simulink model "mech_body_driver"  (Simulink 6.0)
settings: Solver=ode45  StartTime=0.0  StopTime=inf  RelTol=1e-3
libraries: mblibv1 x12
settings Model: Creator=dkennedy  LastModifiedBy=batserve  ExtModeAutoUpdateStatusClock=off
settings DataIOCC: SignalLoggingName=sigsOut
settings OptimizationCC: BooleanDataType=off
settings DebuggingCC: CheckExecutionContextPreStartOutputMsg=on  CheckExecutionContextRuntimeOutputMsg=on  SolverPrmCheckMsg=none
settings HardwareCC: TargetUnknown=on
settings SimMechanicsCC: VisOnUpdateDiagram=on  VisDuringSimulation=on

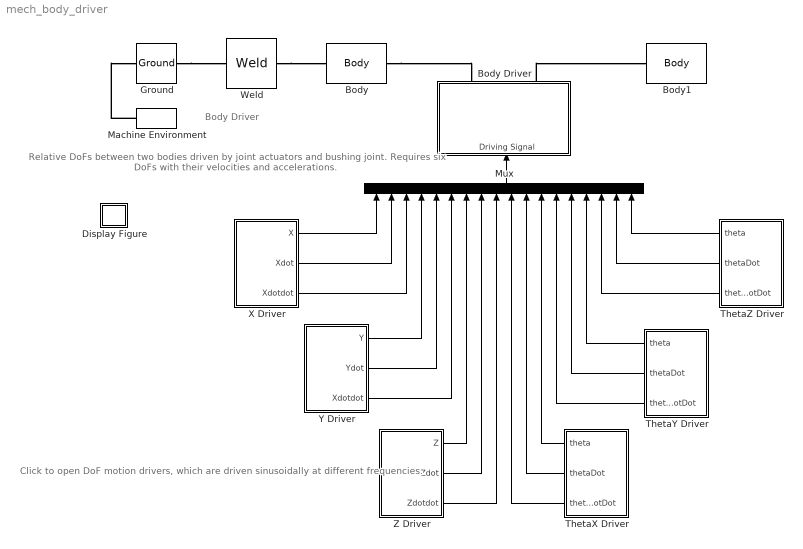
== system mech_body_driver ==
  note: Body Driver
  note: Relative DoFs between two bodies driven by
      | joint actuators and bushing joint. Requires six DoFs with
      | their velocities and accelerations.
  note: Click to open DoF motion drivers,
      | which are driven sinusoidally at
      | different frequencies.
  Body : mblibv1/Bodies/Body  PhysicalDomain=mechanical  SubClassName=Unknown  LeftPortType=workingframe  RightPortType=workingframe  LConnTagsString=CS1  RConnTagsString=CS2  DialogClass=MechanicalBodyBlock  Mass=1  MassUnits=kg  InertiaUnits=kg*m^2  Inertia=0.25*eye(3)  Shape=Cylinder  ShapeDims=[1 1]  ShapeUnits=m  ShapeUse=false  Density=1  DensityUnits=kg/m^3  DensityUse=false  CG=Left$CG$[0 0 0]$WORLD$WORLD$m$[0 0 0]$Euler X-Y-Z$deg$WORLD$false  WorkingFrames=Left$CS1$[0 0 0]$CG$CG$m$[0 0 0]$Euler X-Y-Z$deg$WORLD$true#Right$CS2$[0 0 0]$CG$CG$m$[0 0 0]$Euler X-Y-Z$deg$WORLD$true
  Body Driver : Subsystem  Orientation=up
  Body1 : mblibv1/Bodies/Body  PhysicalDomain=mechanical  SubClassName=Unknown  LeftPortType=workingframe  RightPortType=workingframe  LConnTagsString=CS1  DialogClass=MechanicalBodyBlock  Mass=1  MassUnits=kg  InertiaUnits=kg*m^2  Inertia=[1.5 0 0; 0 1.0 0; 0 0 2.0]  Shape=Cylinder  ShapeDims=[1 1]  ShapeUnits=m  ShapeUse=false  Density=1  DensityUnits=kg/m^3  DensityUse=false  CG=Left$CG$[1 1 1]$WORLD$WORLD$m$[0 0 0]$Euler X-Y-Z$deg$WORLD$false  WorkingFrames=Left$CS1$[0 0 0]$CG$CG$m$[0 0 0]$Euler X-Y-Z$deg$WORLD$true
  Display Figure : Subsystem  Tag=Help  Description="Help callback for body driver model: mech_body_driver.  Opens Help browser to Type 19 marker at documentation for this tutorial model."
      settings: OpenFcn=pmhelpview([docroot '/toolbox/physmod/mech/mech.map'], 'mech_body_driver_help');
      mask Type: Help callback
      mask Display: image(imread('info.bmp'))
  Ground : mblibv1/Bodies/Ground  Opaque=on  LeftPortType=env  RightPortType=workingframe  PhysicalDomain=Mechanical  DialogClass=GroundBlock  CoordPosition=[0 0 0]  CoordPositionUnits=m  StateVectorMgrId=-1  MachineId=[0 0]  ShowEnvPort=on
  Machine Environment : mblibv1/Bodies/Machine Environment  Tag=Factory ground  Orientation=left  DialogController=MECH.DialogSource  Opaque=on  PortType=env  PhysicalDomain=Mechanical  DialogTemplateClass=MECH.MachineEnvironment  SyncWhenCopied=off  Gravity=[0 0 0]  GravityUnits=m/s^2  GravityAsSignal=off  Dimensionality=3D Only  AnalysisType=Forward dynamics  LinearAssemblyTolerance=1e-3  LinearAssemblyToleranceUnits=m  AngularAssemblyTolerance=1e-3  AngularAssemblyToleranceUnits=rad  ConstraintSolverType=Stabilizing  ConstraintRelTolerance=1e-4  ConstraintAbsTolerance=1e-4  UseRobustSingularityHandling=off  StatePerturbationType=Fixed  PerturbationSize=1e-5  VisualizeMachine=on
  Mux : Mux  Orientation=up  Inputs=18
  ThetaX Driver : Subsystem  Orientation=left
  ThetaY Driver : Subsystem  Orientation=left
  ThetaZ Driver : Subsystem  Orientation=left
  Weld : mblibv1/Joints/Weld  PhysicalDomain=mechanical  SubClassName=Unknown  LeftPortType=blob  RightPortType=blob  LConnTagsString=__newl0  RConnTagsString=__newr0  NumSAPorts=0  CutJoint=off  MarkAsCut=off  Primitives=weld  PrimitiveProps=W$INERTIAL$[0 0 0]$weld  DialogClass=JointBlock
  X Driver : Subsystem
  Y Driver : Subsystem
  Z Driver : Subsystem
  wires:
  Mux/1 -> Body Driver/1(Driving Signal)
  X Driver/1(X) -> Mux/1
  X Driver/2(Xdot) -> Mux/2
  X Driver/3(Xdotdot) -> Mux/3
  Y Driver/1(Y) -> Mux/4
  Y Driver/2(Ydot) -> Mux/5
  Y Driver/3(Xdotdot) -> Mux/6
  Z Driver/1(Z) -> Mux/7
  Z Driver/2(Zdot) -> Mux/8
  Z Driver/3(Zdotdot) -> Mux/9
  ThetaX Driver/3(thetaDotDot) -> Mux/10
  ThetaX Driver/2(thetaDot) -> Mux/11
  ThetaX Driver/1(theta) -> Mux/12
  ThetaY Driver/3(thetaDotDot) -> Mux/13
  ThetaY Driver/2(thetaDot) -> Mux/14
  ThetaY Driver/1(theta) -> Mux/15
  ThetaZ Driver/3(thetaDotDot) -> Mux/16
  ThetaZ Driver/2(thetaDot) -> Mux/17
  ThetaZ Driver/1(theta) -> Mux/18
  connections:
  Ground/RConn1 -- Weld/LConn1
  Weld/RConn1 -- Body/LConn1
  Body/RConn1 -- Body Driver/RConn1
  Body Driver/RConn2 -- Body1/LConn1
  Machine Environment/RConn1 -- Ground/LConn1

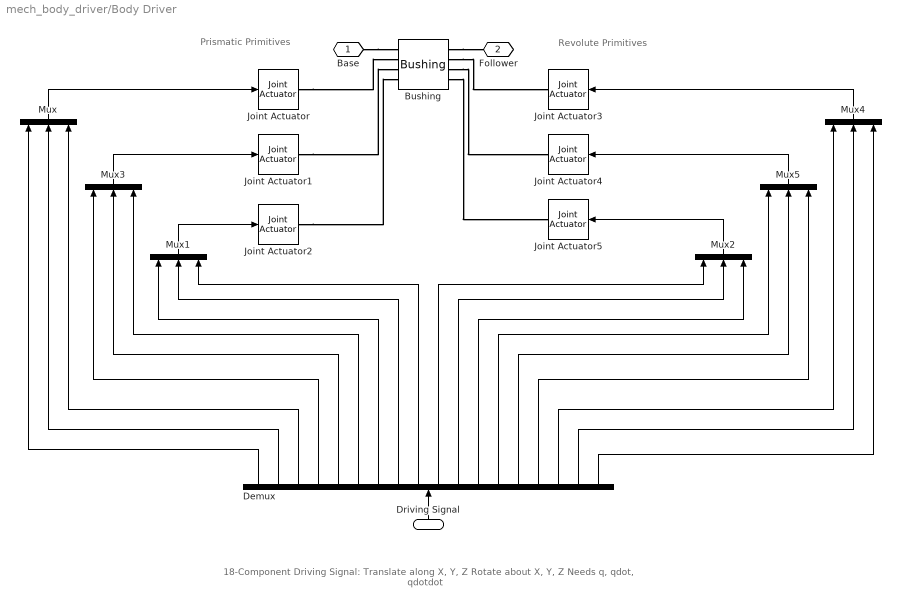
== system mech_body_driver/Body Driver ==
  note: Prismatic Primitives
  note: Revolute Primitives
  note: 18-Component Driving Signal:
      | Translate along X, Y, Z
      | Rotate about X, Y, Z
      | Needs q, qdot, qdotdot
  Driving Signal : Inport  Orientation=up  Port=1  LatchInput=off
  Bushing : mblibv1/Joints/Bushing  PhysicalDomain=mechanical  SubClassName=Unknown  LeftPortType=blob  RightPortType=blob  LConnTagsString=__newl0|SA1|SA2|SA3  RConnTagsString=__newr0|SA1|SA2|SA3  NumSAPorts=6  CutJoint=off  MarkAsCut=off  Primitives=prismatic_prismatic_prismatic_revolute_revolute_revolute  PrimitiveProps=P1$WORLD$[1 0 0]$prismatic#P2$WORLD$[0 1 0]$prismatic#P3$WORLD$[0 0 1]$prismatic#R1$WORLD$[1 0 0]$revolute#R2$WORLD$[0 1 0]$revolute#R3$WORLD$[0 0 1]$revolute  DialogClass=JointBlock
  Demux : Demux  Orientation=up  Outputs=18
  Joint Actuator : mblibv1/Sensors &  Actuators/Joint Actuator  Opaque=on  PhysicalDomain=Mechanical  PortType=blob  ActuationStyle=Motion  AngleUnits=deg  ArcVelocityUnits=deg/s  ArcAccelerationUnits=deg/s^2  CoordPositionUnits=m  VelocityUnits=m/s  AccelerationUnits=m/s^2  ForceUnits=N  TorqueUnits=N-m  ActiveIO=on  Width=3  DialogClass=MechanicalActuatorBlock  Primitive=P1  ReferenceFrame=Absolute (INERTIAL)
  Joint Actuator1 : mblibv1/Sensors &  Actuators/Joint Actuator  Opaque=on  PhysicalDomain=Mechanical  PortType=blob  ActuationStyle=Motion  AngleUnits=deg  ArcVelocityUnits=deg/s  ArcAccelerationUnits=deg/s^2  CoordPositionUnits=m  VelocityUnits=m/s  AccelerationUnits=m/s^2  ForceUnits=N  TorqueUnits=N-m  ActiveIO=on  Width=3  DialogClass=MechanicalActuatorBlock  Primitive=P2  ReferenceFrame=Absolute (INERTIAL)
  Joint Actuator2 : mblibv1/Sensors &  Actuators/Joint Actuator  Opaque=on  PhysicalDomain=Mechanical  PortType=blob  ActuationStyle=Motion  AngleUnits=deg  ArcVelocityUnits=deg/s  ArcAccelerationUnits=deg/s^2  CoordPositionUnits=m  VelocityUnits=m/s  AccelerationUnits=m/s^2  ForceUnits=N  TorqueUnits=N-m  ActiveIO=on  Width=3  DialogClass=MechanicalActuatorBlock  Primitive=P3  ReferenceFrame=Absolute (INERTIAL)
  Joint Actuator3 : mblibv1/Sensors &  Actuators/Joint Actuator  Orientation=left  Opaque=on  PhysicalDomain=Mechanical  PortType=blob  ActuationStyle=Motion  AngleUnits=rad  ArcVelocityUnits=rad/s  ArcAccelerationUnits=rad/s^2  CoordPositionUnits=m  VelocityUnits=m/s  AccelerationUnits=m/s^2  ForceUnits=N  TorqueUnits=N-m  ActiveIO=on  Width=3  DialogClass=MechanicalActuatorBlock  Primitive=R3  ReferenceFrame=Absolute (INERTIAL)
  Joint Actuator4 : mblibv1/Sensors &  Actuators/Joint Actuator  Orientation=left  Opaque=on  PhysicalDomain=Mechanical  PortType=blob  ActuationStyle=Motion  AngleUnits=rad  ArcVelocityUnits=rad/s  ArcAccelerationUnits=rad/s^2  CoordPositionUnits=m  VelocityUnits=m/s  AccelerationUnits=m/s^2  ForceUnits=N  TorqueUnits=N-m  ActiveIO=on  Width=3  DialogClass=MechanicalActuatorBlock  Primitive=R2  ReferenceFrame=Absolute (INERTIAL)
  Joint Actuator5 : mblibv1/Sensors &  Actuators/Joint Actuator  Orientation=left  Opaque=on  PhysicalDomain=Mechanical  PortType=blob  ActuationStyle=Motion  AngleUnits=rad  ArcVelocityUnits=rad/s  ArcAccelerationUnits=rad/s^2  CoordPositionUnits=m  VelocityUnits=m/s  AccelerationUnits=m/s^2  ForceUnits=N  TorqueUnits=N-m  ActiveIO=on  Width=3  DialogClass=MechanicalActuatorBlock  Primitive=R1  ReferenceFrame=Absolute (INERTIAL)
  Mux{,1..5} (6 alike) : Mux  Orientation=up  Inputs=3
  Base : PMIOPort  Port=1  Side=Right
  Follower : PMIOPort  Orientation=left  Port=2  Side=Right
  wires:
  Mux/1 -> Joint Actuator/1
  Mux1/1 -> Joint Actuator2/1
  Mux4/1 -> Joint Actuator3/1
  Mux5/1 -> Joint Actuator4/1
  Mux2/1 -> Joint Actuator5/1
  Driving Signal/1 -> Demux/1
  Mux3/1 -> Joint Actuator1/1
  Demux/1 -> Mux/1
  Demux/2 -> Mux/2
  Demux/3 -> Mux/3
  Demux/4 -> Mux3/1
  Demux/5 -> Mux3/2
  Demux/6 -> Mux3/3
  Demux/7 -> Mux1/1
  Demux/8 -> Mux1/2
  Demux/9 -> Mux1/3
  Demux/10 -> Mux2/1
  Demux/11 -> Mux2/2
  Demux/12 -> Mux2/3
  Demux/13 -> Mux5/1
  Demux/14 -> Mux5/2
  Demux/15 -> Mux5/3
  Demux/16 -> Mux4/1
  Demux/17 -> Mux4/2
  Demux/18 -> Mux4/3
  connections:
  Bushing/RConn1 -- Follower/RConn1
  Base/RConn1 -- Bushing/LConn1
  Joint Actuator/RConn1 -- Bushing/LConn2
  Joint Actuator2/RConn1 -- Bushing/LConn4
  Joint Actuator1/RConn1 -- Bushing/LConn3
  Bushing/RConn2 -- Joint Actuator3/RConn1
  Bushing/RConn3 -- Joint Actuator4/RConn1
  Bushing/RConn4 -- Joint Actuator5/RConn1

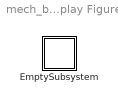
== system mech_body_driver/Display Figure ==
  EmptySubsystem : Subsystem

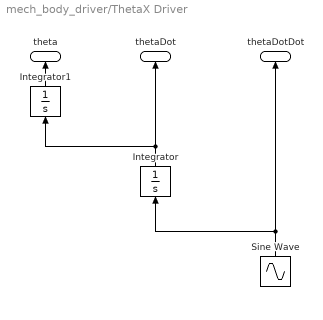
== system mech_body_driver/ThetaX Driver ==
  Integrator : Integrator  Orientation=up
  Integrator1 : Integrator  Orientation=up
  Sine Wave : Sin  Orientation=up  Amplitude=-(pi/4)*(2*pi/16)^2  Frequency=2*pi/16  Phase=pi/2  SampleTime=0
  theta : Outport  Orientation=up
  thetaDot : Outport  Orientation=up  Port=2
  thetaDotDot : Outport  Orientation=up  Port=3
  wires:
  Integrator/1 -> thetaDot/1, Integrator1/1
  Sine Wave/1 -> thetaDotDot/1, Integrator/1
  Integrator1/1 -> theta/1

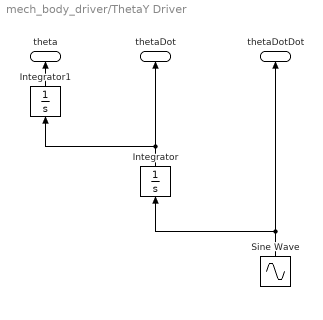
== system mech_body_driver/ThetaY Driver ==
  Integrator : Integrator  Orientation=up
  Integrator1 : Integrator  Orientation=up
  Sine Wave : Sin  Orientation=up  Amplitude=-(pi/4)*(2*pi/8)^2  Frequency=2*pi/8  Phase=pi/2  SampleTime=0
  theta : Outport  Orientation=up
  thetaDot : Outport  Orientation=up  Port=2
  thetaDotDot : Outport  Orientation=up  Port=3
  wires:
  Integrator/1 -> thetaDot/1, Integrator1/1
  Sine Wave/1 -> thetaDotDot/1, Integrator/1
  Integrator1/1 -> theta/1

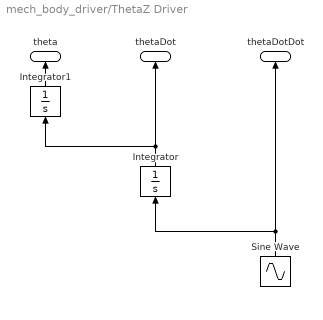
== system mech_body_driver/ThetaZ Driver ==
  Integrator : Integrator  Orientation=up
  Integrator1 : Integrator  Orientation=up
  Sine Wave : Sin  Orientation=up  Amplitude=-(pi/4)*(2*pi/4)^2  Frequency=2*pi/4  Phase=pi/2  SampleTime=0
  theta : Outport  Orientation=up
  thetaDot : Outport  Orientation=up  Port=2
  thetaDotDot : Outport  Orientation=up  Port=3
  wires:
  Integrator/1 -> thetaDot/1, Integrator1/1
  Sine Wave/1 -> thetaDotDot/1, Integrator/1
  Integrator1/1 -> theta/1

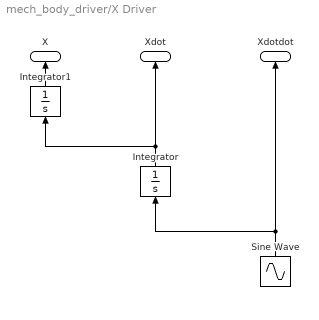
== system mech_body_driver/X Driver ==
  Integrator : Integrator  Orientation=up
  Integrator1 : Integrator  Orientation=up
  Sine Wave : Sin  Orientation=up  Amplitude=-1.0*(2*pi/32)^2  Frequency=2*pi/32  Phase=pi/2  SampleTime=0
  X : Outport  Orientation=up
  Xdot : Outport  Orientation=up  Port=2
  Xdotdot : Outport  Orientation=up  Port=3
  wires:
  Integrator1/1 -> X/1
  Sine Wave/1 -> Integrator/1, Xdotdot/1
  Integrator/1 -> Integrator1/1, Xdot/1

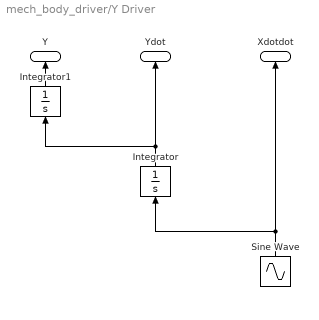
== system mech_body_driver/Y Driver ==
  Integrator : Integrator  Orientation=up
  Integrator1 : Integrator  Orientation=up
  Sine Wave : Sin  Orientation=up  Amplitude=-1.0*(2*pi/16)^2  Frequency=2*pi/16  Phase=pi/2  SampleTime=0
  Y : Outport  Orientation=up
  Ydot : Outport  Orientation=up  Port=2
  Xdotdot : Outport  Orientation=up  Port=3
  wires:
  Integrator/1 -> Ydot/1, Integrator1/1
  Sine Wave/1 -> Xdotdot/1, Integrator/1
  Integrator1/1 -> Y/1

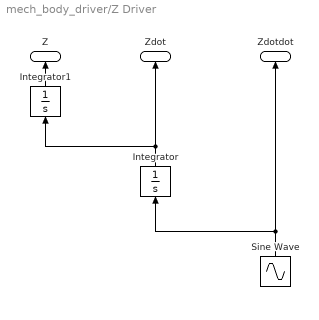
== system mech_body_driver/Z Driver ==
  Integrator : Integrator  Orientation=up
  Integrator1 : Integrator  Orientation=up
  Sine Wave : Sin  Orientation=up  Amplitude=-1.0*(2*pi/4)^2  Frequency=2*pi/4  Phase=pi/2  SampleTime=0
  Z : Outport  Orientation=up
  Zdot : Outport  Orientation=up  Port=2
  Zdotdot : Outport  Orientation=up  Port=3
  wires:
  Integrator/1 -> Zdot/1, Integrator1/1
  Sine Wave/1 -> Zdotdot/1, Integrator/1
  Integrator1/1 -> Z/1

== system mech_body_driver/Display Figure/EmptySubsystem ==
